simulink model "planta"  (R2021b)
settings: Solver=FixedStepAuto  StartTime=0.0  StopTime=20  FixedStep=0.00001  RelTol=1e-3
undefined symbols (not defined in the file): b, d1, d2, Gden, Gnum, I, k, pwm, timeR, wb, wcp, wm
libraries: simulink x2
settings Model: Creator=felip  LastModifiedBy=felip

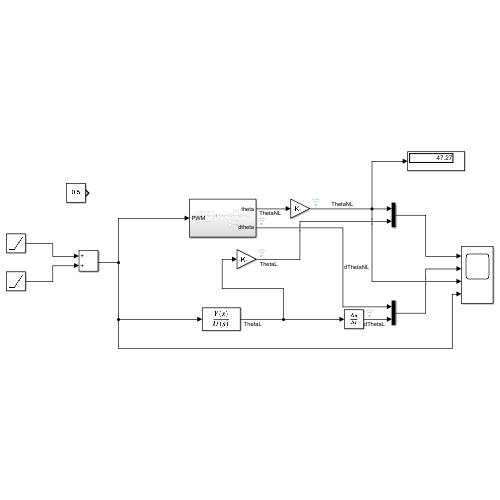
[thumbnail: Simulink's stored preview of the top-level diagram]
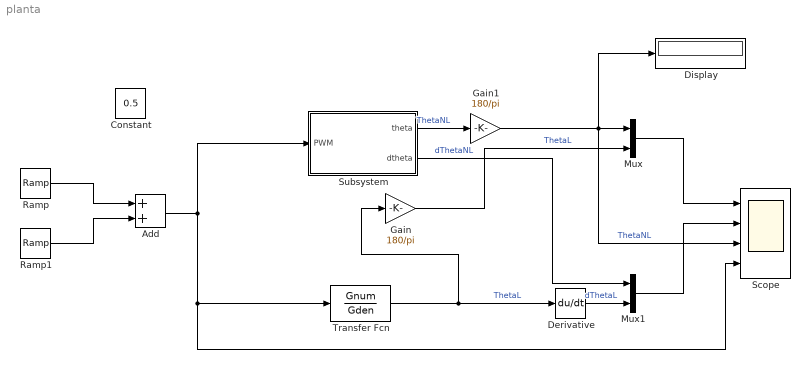
== system planta ==
  Add : Sum
  Constant : Constant  Value=0.5
  Derivative : Derivative
  Display : Display
  Gain : Gain  Gain=180/pi
  Gain1 : Gain  Gain=180/pi
  Mux : Mux  Inputs=2
  Mux1 : Mux  Inputs=2
  Ramp : simulink/Sources/Ramp  slope=pwm/timeR  start=0  InitialOutput=0
  Ramp1 : simulink/Sources/Ramp  slope=-pwm/timeR  start=timeR  InitialOutput=0
  Scope : Scope  NumInputPorts=4
  Subsystem : Subsystem
  Transfer Fcn : TransferFcn  Numerator=Gnum  Denominator=Gden
  wires:
  Transfer Fcn/1 -> Gain/1, Derivative/1  "ThetaL"
  Derivative/1 -> Mux1/2  "dThetaL"
  Subsystem/2(dtheta) -> Mux1/1  "dThetaNL"
  Subsystem/1(theta) -> Gain1/1  "ThetaNL"
  Mux1/1 -> Scope/2
  Add/1 -> Transfer Fcn/1, Scope/4, Subsystem/1(PWM)
  Gain/1 -> Mux/2  "ThetaL"
  Mux/1 -> Scope/1
  Gain1/1 -> Display/1, Scope/3, Mux/1  "ThetaNL"
  Ramp/1 -> Add/1
  Ramp1/1 -> Add/2

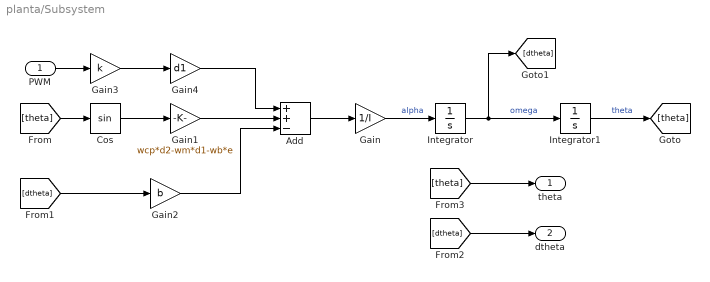
== system planta/Subsystem ==
  PWM : Inport
  Add : Sum  Inputs=++-
  Cos : Trigonometry
  Gain : Gain  Gain=1/I
  Gain1 : Gain  Gain=wcp*d2-wm*d1-wb*e
  Gain2 : Gain  Gain=b
  Gain3 : Gain  Gain=k
  Gain4 : Gain  Gain=d1
  Integrator : Integrator
  Integrator1 : Integrator
  theta : Outport
  dtheta : Outport  Port=2
  wires:
  Gain2/1 -> Add/3
  Gain/1 -> Integrator/1  "alpha"
  Integrator/1 -> [dtheta], Integrator1/1  "omega"
  Integrator1/1 -> [theta]  "theta"
  Add/1 -> Gain/1
  Cos/1 -> Gain1/1
  Gain1/1 -> Add/2
  [theta] -> Cos/1
  [theta] -> theta/1
  [dtheta] -> Gain2/1
  PWM/1 -> Gain3/1
  [dtheta] -> dtheta/1
  Gain4/1 -> Add/1
  Gain3/1 -> Gain4/1
